simulink model "base_control_object"  (R2021b)
settings: Solver=VariableStepAuto  StartTime=0.0  StopTime=10.0  RelTol=1e-3
values from neighbouring files (symbols this model uses):
  C12 = C12_nom*Y(3)    [compare_tf_coeffs_dispersion.m]
  J1 = J1_nom*Y(1)    [compare_tf_coeffs_dispersion.m]
  J2 = J2_nom*Y(2)    [compare_tf_coeffs_dispersion.m]
  Kd = Kd_nom*Y(4)    [compare_tf_coeffs_dispersion.m]
undefined symbols (not defined in the file or in its folder): C, Ksp, Ra, Ta
settings Model: Creator=Ilya  LastModifiedBy=Ilya

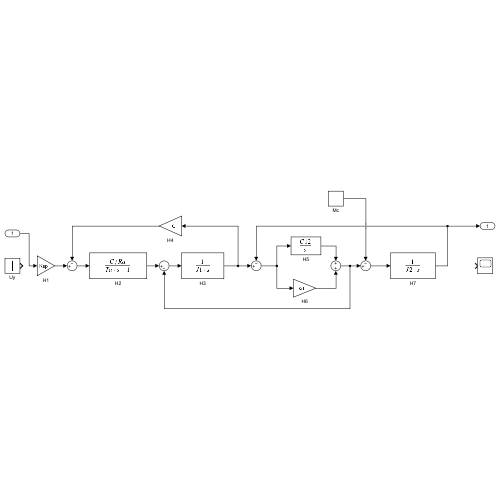
[thumbnail: Simulink's stored preview of the top-level diagram]
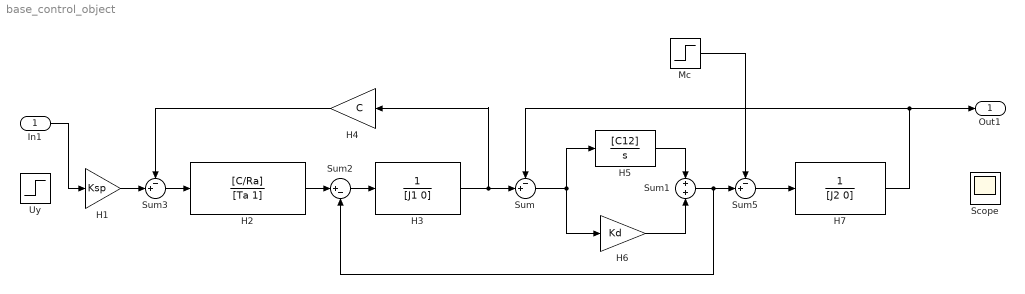
== system base_control_object ==
  In1 : Inport
  H1 : Gain  Gain=Ksp
  H2 : TransferFcn  Numerator=[C/Ra]  Denominator=[Ta 1]
  H3 : TransferFcn  Denominator=[J1 0]
  H4 : Gain  Gain=C
  H5 : TransferFcn  Numerator=[C12]  Denominator=[1 0]
  H6 : Gain  Gain=Kd
  H7 : TransferFcn  Denominator=[J2 0]
  Mc : Step  Time=5  After=10  SampleTime=0
  Scope : Scope
  Sum : Sum  Inputs=-+|
  Sum1 : Sum  Inputs=+|+
  Sum2 : Sum  Inputs=|+-
  Sum3 : Sum  Inputs=-+|
  Sum5 : Sum  Inputs=-+|
  Uy : Step  Time=0  After=10  SampleTime=0
  Out1 : Outport
  wires:
  Sum/1 -> H6/1, H5/1
  H7/1 -> Out1/1, Sum/1
  H5/1 -> Sum1/1
  Sum2/1 -> H3/1
  H6/1 -> Sum1/2
  H1/1 -> Sum3/2
  H2/1 -> Sum2/1
  Sum5/1 -> H7/1
  Sum1/1 -> Sum5/2, Sum2/2
  H3/1 -> H4/1, Sum/2
  Mc/1 -> Sum5/1
  H4/1 -> Sum3/1
  Sum3/1 -> H2/1
  In1/1 -> H1/1
